simulink model "controller"  (R2023a)
settings: Solver=VariableStepAuto  StartTime=0.0  StopTime=10.0  RelTol=1e-3
values from neighbouring files (symbols this model uses):
  b_control = T(speed,3)    [MAIN_Protocol_Simulation.m]    (also in find_fluid_profile.m)
  c_start = VP_Inputs.ind_CL_start*Dt    [MAIN_Protocol_Simulation.m]
  Ki_control = T(speed,2)    [MAIN_Protocol_Simulation.m]    (also in find_fluid_profile.m)
  Kp_control = T(speed,1)    [MAIN_Protocol_Simulation.m]    (also in find_fluid_profile.m)
  target = DATASET{1,sidx}.Controller_Target    [MAIN_Protocol_Simulation.m]
  u_max = 2000    [MAIN_Protocol_Simulation.m]    (also in controller_discrete_time.m; find_fluid_profile.m)
settings Model: Creator=yekanth  LastModifiedBy=yekanth

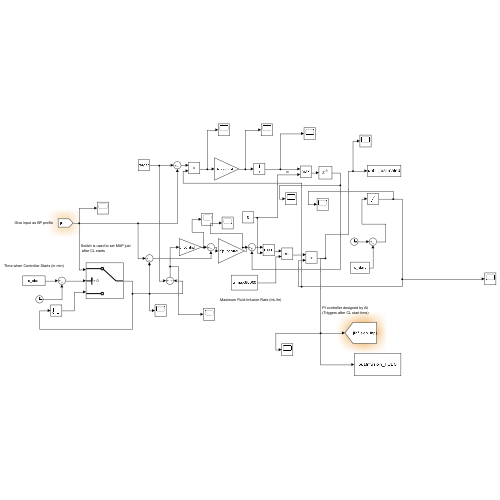
[thumbnail: Simulink's stored preview of the top-level diagram]
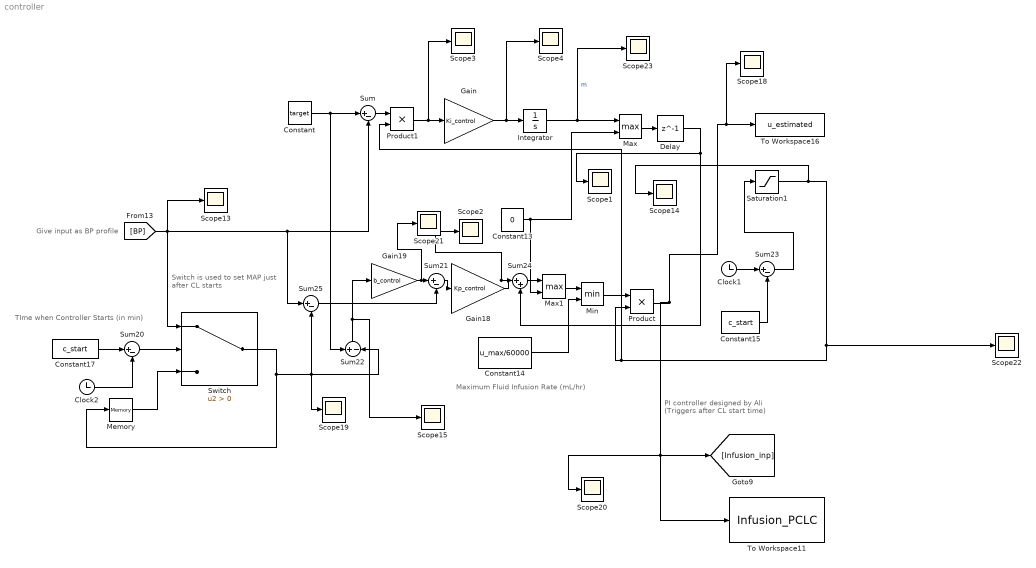
== system controller ==
  note: TIme when Controller Starts (in min)
  note: PI controller designed by Ali
      | (Triggers after CL start time)
  note: Switch is used to set MAP just
      |  after CL starts
  note: Maximum Fluid Infusion Rate (mL/hr)
  note: Give input as BP profile
  Clock1 : Clock
  Clock2 : Clock
  Constant : Constant  Value=target
  Constant13 : Constant  Value=0
  Constant14 : Constant  Value=u_max/60000
  Constant15 : Constant  Value=c_start
  Constant17 : Constant  Value=c_start
  Delay : Delay  DelayLength=1  InitialCondition=0
  Gain : Gain  Gain=Ki_control
  Gain18 : Gain  Gain=Kp_control
  Gain19 : Gain  Gain=b_control
  Integrator : Integrator
  Max : MinMax  Function=max  Inputs=2
  Max1 : MinMax  Function=max  Inputs=2
  Memory : Memory
  Min : MinMax  Inputs=2
  Product : Product
  Product1 : Product
  Saturation1 : Saturate  UpperLimit=1  LowerLimit=0
  Scope{1..4,13..15,18..23} (13 alike) : Scope
  Sum{,20..21,23,25} (5 alike) : Sum  Inputs=|+-
  Sum22 : Sum  Inputs=+-
  Sum24 : Sum  Inputs=|++
  Switch : Switch  Criteria=u2 > Threshold  SaturateOnIntegerOverflow=off  InputSameDT=off
  To Workspace11 : ToWorkspace  VariableName=Infusion_PCLC  SampleTime=-1
  To Workspace16 : ToWorkspace  VariableName=u_estimated  SaveFormat=Timeseries  SampleTime=-1
  wires:
  [BP] -> Scope13/1, Sum25/1, Sum/2, Switch/1
  Min/1 -> Product/1
  Clock2/1 -> Sum20/2
  Gain19/1 -> Scope21/1, Sum21/1
  Max/1 -> Delay/1
  Sum24/1 -> Max1/1
  Constant17/1 -> Sum20/1
  Clock1/1 -> Sum23/1
  Delay/1 -> Scope1/1, Sum24/2
  Sum25/1 -> Sum21/2
  Sum21/1 -> Gain18/1
  Constant/1 -> Sum/1, Sum22/1
  Sum20/1 -> Switch/2
  Constant13/1 -> Max/2, Max1/2
  Constant15/1 -> Sum23/2
  Product1/1 -> Scope3/1, Gain/1
  Switch/1 -> Scope19/1, Sum25/2, Sum22/2, Memory/1
  Memory/1 -> Switch/3
  Gain/1 -> Scope4/1, Integrator/1
  Sum23/1 -> Saturation1/1
  Integrator/1 -> Scope23/1, Max/1  "m"
  Saturation1/1 -> Scope14/1, Product1/2, Product/2, Scope22/1
  Max1/1 -> Min/1
  Sum22/1 -> Scope15/1, Gain19/1
  Gain18/1 -> Scope2/1, Sum24/1
  Constant14/1 -> Min/2
  Product/1 -> [Infusion_inp], Scope20/1, To Workspace11/1, Scope18/1, To Workspace16/1
  Sum/1 -> Product1/1
